simulink model "Vehicle_trailer_FreeModelControl"  (R2015a)
settings: Solver=ode3  StartTime=0.0  StopTime=30.0  FixedStep=Ts  RelTol=1e-3
undefined symbols (not defined in the file): alfa1, BWbaja, Df, jkk, kdf, kif, kpf, L1, L12, L2, manuever, tolerance, Ts, v
settings Model: Creator=Sara  LastModifiedBy=Sara
settings DebuggingCC: FcnCallInpInsideContextMsg=EnableAllAsWarning
settings GRTTargetCC: CombineOutputUpdateFcns=off  GRTInterface=on

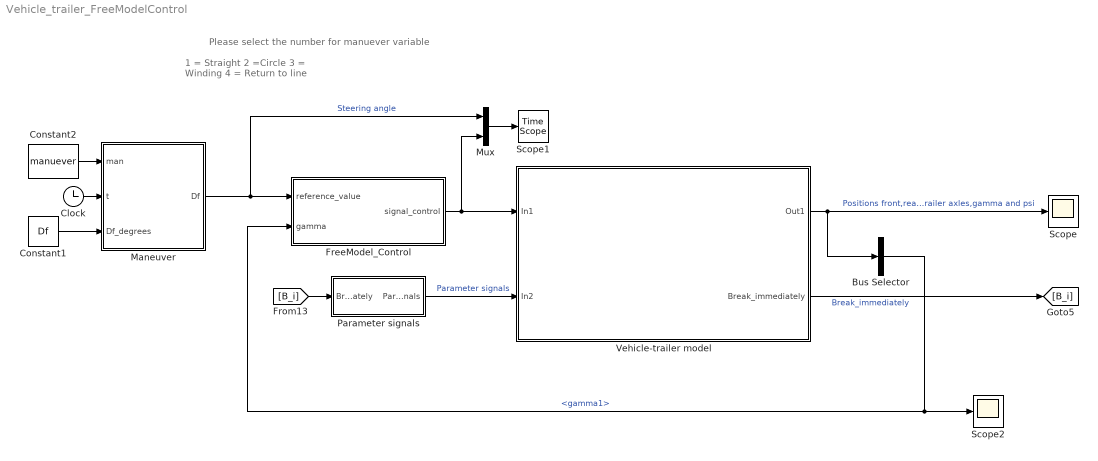
== system Vehicle_trailer_FreeModelControl ==
  note: 1 = Straight
      | 2 =Circle
      | 3 = Winding
      | 4 = Return to line
  note: Please select the number for manuever variable
  Bus Selector : BusSelector  OutputSignals=gamma1
  Clock : Clock
  Constant1 : Constant  Value=Df
  Constant2 : Constant  Value=manuever
  FreeModel_Control : Subsystem
  Maneuver : MATLAB Function  TreatAsAtomicUnit=on
  Mux : Mux  Inputs=2
  Parameter signals : Subsystem
  Scope : Scope
      settings: YMin=-15.4299  YMax=114.11
  Scope1 : TimeScope
  Scope2 : Scope
      settings: YMin=-15.4299  YMax=114.11  SaveName=ScopeData_SteeringAngle1
  Vehicle-trailer model : Subsystem
      mask Display: image(imread('vt.png'))
  wires:
  Constant2/1 -> Maneuver/1(man)
  Clock/1 -> Maneuver/2(t)
  Vehicle-trailer model/1(Out1) -> Scope/1, Bus Selector/1  "Positions front,rear and trailer axles,gamma and psi"
  Parameter signals/1(Parameter signals) -> Vehicle-trailer model/2(In2)  "Parameter signals"
  Vehicle-trailer model/2(Break_immediately) -> [B_i]  "Break_immediately"
  [B_i] -> Parameter signals/1(Break_immediately)
  Constant1/1 -> Maneuver/3(Df_degrees)
  Maneuver/1(Df) -> Mux/1, FreeModel_Control/1(reference_value)  "Steering angle"
  Bus Selector/1 -> Scope2/1, FreeModel_Control/2(gamma)  "<gamma1>"
  FreeModel_Control/1(signal_control) -> Mux/2, Vehicle-trailer model/1(In1)
  Mux/1 -> Scope1/1

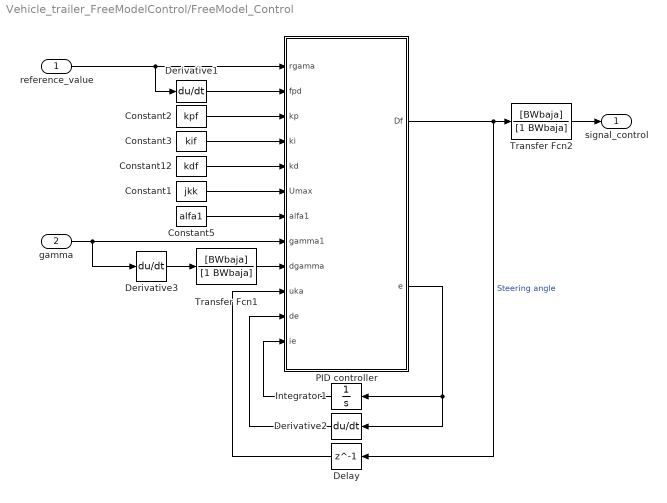
== system Vehicle_trailer_FreeModelControl/FreeModel_Control ==
  reference_value : Inport
  gamma : Inport  Port=2
  Constant1 : Constant  Value=jkk
  Constant12 : Constant  Value=kdf
  Constant2 : Constant  Value=kpf
  Constant3 : Constant  Value=kif
  Constant5 : Constant  Value=alfa1
  Delay : Delay  DelayLength=1  InitialCondition=0  SampleTime=Ts
  Derivative1 : Derivative
  Derivative2 : Derivative
  Derivative3 : Derivative
  Integrator1 : Integrator
  PID controller : MATLAB Function  TreatAsAtomicUnit=on
  Transfer Fcn1 : TransferFcn  Numerator=[BWbaja]  Denominator=[1 BWbaja]
  Transfer Fcn2 : TransferFcn  Numerator=[BWbaja]  Denominator=[1 BWbaja]
  signal_control : Outport
  wires:
  Derivative1/1 -> PID controller/2(fpd)
  Constant2/1 -> PID controller/3(kp)
  Constant3/1 -> PID controller/4(ki)
  PID controller/2(e) -> Derivative2/1, Integrator1/1
  Constant5/1 -> PID controller/7(alfa1)
  Delay/1 -> PID controller/10(uka)
  Integrator1/1 -> PID controller/12(ie)
  Derivative2/1 -> PID controller/11(de)
  PID controller/1(Df) -> Transfer Fcn2/1, Delay/1  "Steering angle"
  Constant12/1 -> PID controller/5(kd)
  reference_value/1 -> PID controller/1(rgama), Derivative1/1
  Derivative3/1 -> Transfer Fcn1/1
  Transfer Fcn1/1 -> PID controller/9(dgamma)
  gamma/1 -> Derivative3/1, PID controller/8(gamma1)
  Constant1/1 -> PID controller/6(Umax)
  Transfer Fcn2/1 -> signal_control/1

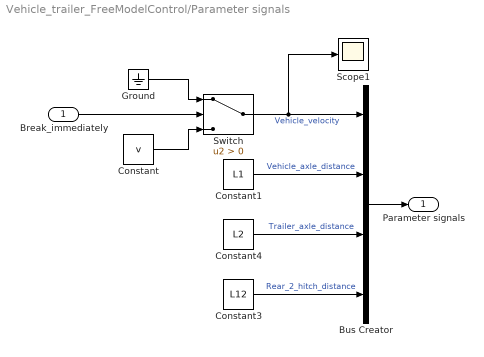
== system Vehicle_trailer_FreeModelControl/Parameter signals ==
  Break_immediately : Inport
  Bus Creator : BusCreator
  Constant : Constant  Value=v
  Constant1 : Constant  Value=L1
  Constant3 : Constant  Value=L12
  Constant4 : Constant  Value=L2
  Ground : Ground
  Scope1 : Scope
      settings: YMin=-1  YMax=1  SaveName=ScopeData4
  Switch : Switch  Criteria=u2 > Threshold
  Parameter signals : Outport
  wires:
  Constant1/1 -> Bus Creator/2  "Vehicle_axle_distance"
  Constant4/1 -> Bus Creator/3  "Trailer_axle_distance"
  Constant3/1 -> Bus Creator/4  "Rear_2_hitch_distance"
  Bus Creator/1 -> Parameter signals/1
  Switch/1 -> Bus Creator/1, Scope1/1  "Vehicle_velocity"
  Break_immediately/1 -> Switch/2
  Ground/1 -> Switch/1
  Constant/1 -> Switch/3

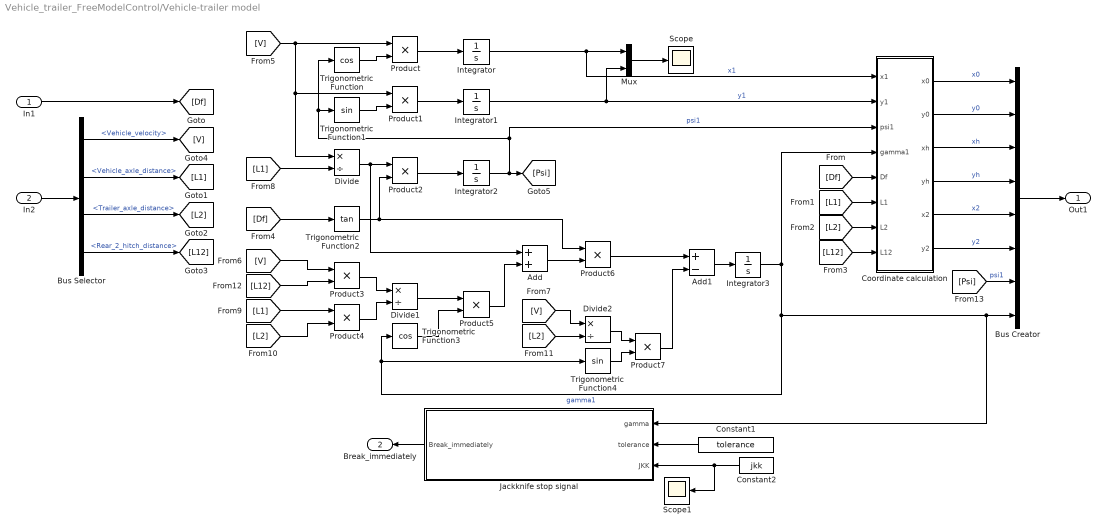
== system Vehicle_trailer_FreeModelControl/Vehicle-trailer model ==
  In1 : Inport
  In2 : Inport  Port=2
  Add : Sum
  Add1 : Sum  Inputs=+-
  Bus Creator : BusCreator  Inputs=8
  Bus Selector : BusSelector  OutputSignals=Vehicle_velocity,Vehicle_axle_distance,Trailer_axle_distance,Rear_2_hitch_distance
  Constant1 : Constant  Value=tolerance
  Constant2 : Constant  Value=jkk
  Coordinate calculation : MATLAB Function  TreatAsAtomicUnit=on
  Divide : Product  Inputs=*/
  Divide1 : Product  Inputs=*/
  Divide2 : Product  Inputs=*/
  Integrator{,1..3} (4 alike) : Integrator
  "Jackknife stop signal " : MATLAB Function  TreatAsAtomicUnit=on
  Mux : Mux  Inputs=2
  Product{,1..7} (8 alike) : Product
  Scope : Scope
      settings: YMin=-15.0157  YMax=26.5952  SaveName=Car
  Scope1 : Scope
      settings: YMin=-15.0157  YMax=26.5952  SaveName=ScopeData_jkk
  Trigonometric Function : Trigonometry  Operator=cos
  Trigonometric Function1 : Trigonometry
  Trigonometric Function2 : Trigonometry  Operator=tan
  Trigonometric Function3 : Trigonometry  Operator=cos
  Trigonometric Function4 : Trigonometry
  Out1 : Outport
  Break_immediately : Outport  Port=2
  wires:
  Trigonometric Function4/1 -> Product7/2
  Divide2/1 -> Product7/1
  Trigonometric Function1/1 -> Product1/2
  Product1/1 -> Integrator1/1
  Trigonometric Function3/1 -> Product5/2
  Product2/1 -> Integrator2/1
  Divide/1 -> Product2/1, Add/1
  Trigonometric Function2/1 -> Product6/1, Product2/2
  Product6/1 -> Add1/1
  Add1/1 -> Integrator3/1
  Divide1/1 -> Product5/1
  Integrator3/1 -> Trigonometric Function4/1, Trigonometric Function3/1, Bus Creator/8, "Jackknife stop signal "/1(gamma), Coordinate calculation/4(gamma1)  "gamma1"
  Product7/1 -> Add1/2
  Add/1 -> Product6/2
  Product3/1 -> Divide1/1
  Integrator2/1 -> [Psi], Trigonometric Function/1, Trigonometric Function1/1, Coordinate calculation/3(psi1)  "psi1"
  Trigonometric Function/1 -> Product/2
  Product5/1 -> Add/2
  Product4/1 -> Divide1/2
  Product/1 -> Integrator/1
  Integrator/1 -> Coordinate calculation/1(x1), Mux/1  "x1"
  Integrator1/1 -> Mux/2, Coordinate calculation/2(y1)  "y1"
  Mux/1 -> Scope/1
  Bus Creator/1 -> Out1/1
  [Df] -> Coordinate calculation/5(Df)
  [L1] -> Coordinate calculation/6(L1)
  [L2] -> Coordinate calculation/7(L2)
  [L12] -> Coordinate calculation/8(L12)
  [Df] -> Trigonometric Function2/1
  [V] -> Divide/1, Product1/1, Product/1
  [V] -> Product3/1
  [V] -> Divide2/1
  [L1] -> Divide/2
  [L1] -> Product4/1
  [L2] -> Product4/2
  [L2] -> Divide2/2
  [L12] -> Product3/2
  Coordinate calculation/1(x0) -> Bus Creator/1  "x0"
  Coordinate calculation/2(y0) -> Bus Creator/2  "y0"
  [Psi] -> Bus Creator/7  "psi1"
  Coordinate calculation/3(xh) -> Bus Creator/3  "xh"
  Coordinate calculation/4(yh) -> Bus Creator/4  "yh"
  Coordinate calculation/5(x2) -> Bus Creator/5  "x2"
  Coordinate calculation/6(y2) -> Bus Creator/6  "y2"
  In2/1 -> Bus Selector/1
  Bus Selector/1 -> [V]  "<Vehicle_velocity>"
  Bus Selector/2 -> [L1]  "<Vehicle_axle_distance>"
  Bus Selector/3 -> [L2]  "<Trailer_axle_distance>"
  Bus Selector/4 -> [L12]  "<Rear_2_hitch_distance>"
  In1/1 -> [Df]
  "Jackknife stop signal "/1(Break_immediately) -> Break_immediately/1
  Constant1/1 -> "Jackknife stop signal "/2(tolerance)
  Constant2/1 -> Scope1/1, "Jackknife stop signal "/3(JKK)

== matlab function Vehicle_trailer_FreeModelControl/Maneuver ==
  data: man input; Df output; t input; Df_degrees input
function Df = fcn(man,t,Df_degrees)

switch man
    case 1
        Df=0;
    case 2
        Df=Df_degrees*pi/180;
    case 3
        if t<5
            Df=0;
        elseif (t>=5) && (t<10)
            Df=Df_degrees*pi/180;
        elseif (t>=10) && (t<15)
            Df=0;
        elseif (t>=15) && (t<20)
            Df=-Df_degrees*pi/180;
        elseif (t>=20) && (t<25)
            Df=0;
        else
            Df=Df_degrees*pi/180;
        end
    case 4
        if t<5
            Df=0;
        elseif (t>=5) && (t<10)
            Df=Df_degrees*pi/180;
        else
            Df=0;
        end
    otherwise
        Df=0;
end

== matlab function Vehicle_trailer_FreeModelControl/Vehicle-trailer model/Coordinate calculation ==
  data: x1 input; x0 output; y1 input; psi1 input; gamma1 input; Df input; L1 input; L2 input; L12 input; y0 output; xh output; yh output; x2 output; y2 output
function [x0,y0,xh,yh,x2,y2] = fcn(x1,y1,psi1,gamma1,Df,L1,L2,L12)
psi2=psi1-gamma1;
psi0=psi1+Df;

x0=x1+L1*cos(psi1);
y0=y1+L1*sin(psi1);
xh=x1-L12*cos(psi1);
yh=y1-L12*sin(psi1);
x2=x1-L12*cos(psi1)-L2*cos(psi2);
y2=y1-L12*sin(psi1)-L2*sin(psi2);

== matlab function Vehicle_trailer_FreeModelControl/Vehicle-trailer model/Jackknife stop signal  ==
  data: gamma input; tolerance input; Break_immediately output; JKK input
function Break_immediately = fcn(gamma,tolerance,JKK)
%#codegen

if abs(gamma) > tolerance*JKK 
    Break_immediately=1;
else
    Break_immediately=0;
end

== matlab function Vehicle_trailer_FreeModelControl/FreeModel_Control/PID controller ==
  data: rgama input; fpd input; kp input; ki input; kd input; Umax input; alfa1 input; gamma1 input; dgamma input; uka input; de input; Df output; e output; ie input
function [Df,e]= fcn(rgama,fpd,kp,ki,kd,Umax,alfa1,gamma1,dgamma,uka,de,ie)
Fe=dgamma-alfa1*uka;
e=rgama-gamma1;
upi=kp*e+ki*ie+kd*de;
u=((Fe-fpd)+upi)*1/alfa1;
if abs(u)>Umax
    Df=Umax*sign(u);
else
    Df=u;
end
